simulink library "csu_ftc_final_thruster_cmd_mtv_lib"  (R2014b)
settings: Solver=ode45  StartTime=0.0  StopTime=10.0  RelTol=1e-3
undefined symbols (not defined in the file or in its folder): act_acs_cmd_duration_bias, coarse10_time, coarse11_time, coarse12_time, coarse1_time, coarse2_time, coarse3_time, coarse4_time, coarse5_time, coarse6_time, coarse7_time, coarse8_time, coarse9_time, fsw_dt
libraries: simulink x4, util_event_lib x3, util_info_lib x1
settings Model: Creator=escrane  LastModifiedBy=tgorton

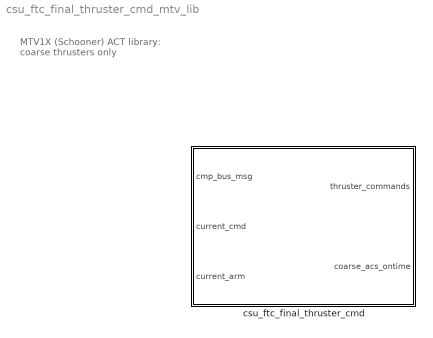
== system csu_ftc_final_thruster_cmd_mtv_lib ==
  note: MTV1X (Schooner) ACT library:
      | coarse thrusters only
  " csu_ftc_final_thruster_cmd" : Subsystem

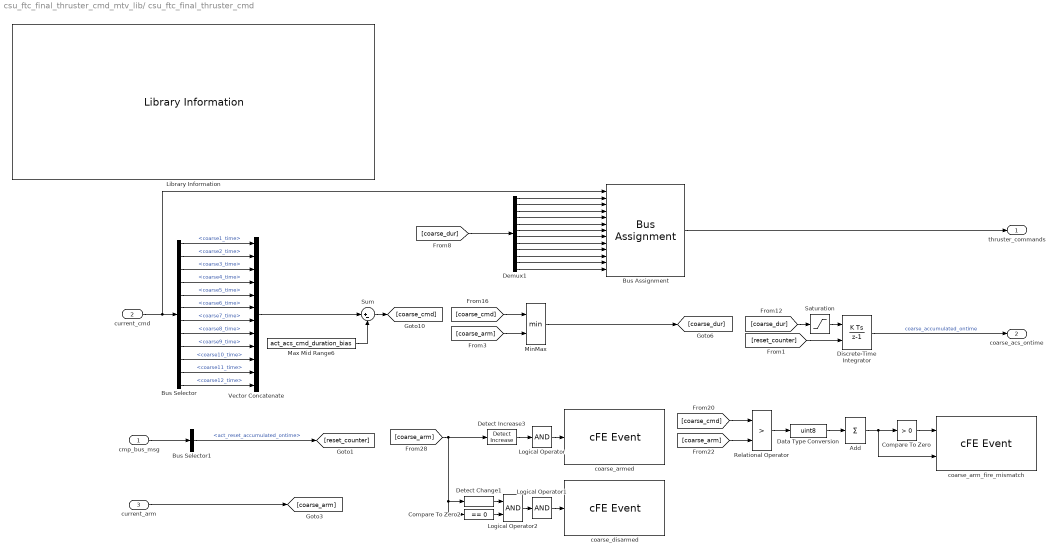
== system csu_ftc_final_thruster_cmd_mtv_lib/ csu_ftc_final_thruster_cmd ==
  cmp_bus_msg : Inport
  current_cmd : Inport  Port=2
  current_arm : Inport  Port=3
  Add : Sum  Inputs=+
  Bus Assignment : BusAssignment  AssignedSignals=coarse1_time,coarse2_time,coarse3_time,coarse4_time,coarse5_time,coarse6_time,coarse7_time,coarse8_time,coarse9_time,coarse10_time,coarse11_time,coarse12_time
  Bus Selector : BusSelector  OutputSignals=coarse1_time,coarse2_time,coarse3_time,coarse4_time,coarse5_time,coarse6_time,coarse7_time,coarse8_time,coarse9_time,coarse10_time,coarse11_time,coarse12_time
  Bus Selector1 : BusSelector  OutputSignals=act_reset_accumulated_ontime
  Compare To Zero : simulink/Logic and Bit Operations/Compare To Zero  relop=>  OutDataTypeStr=boolean
  Compare To Zero2 : simulink/Logic and Bit Operations/Compare To Zero  relop===  OutDataTypeStr=boolean
  Data Type Conversion : DataTypeConversion  OutDataTypeStr=uint8
  Demux1 : Demux  Outputs=12
  Detect Change1 : simulink/Logic and Bit Operations/Detect Change  vinit=0  InputProcessing=Inherited  OutDataTypeStr=boolean
  Detect Increase3 : simulink/Logic and Bit Operations/Detect Increase  vinit=0.0  InputProcessing=Inherited  OutDataTypeStr=boolean
  Discrete-Time Integrator : DiscreteIntegrator  gainval=1/fsw_dt  ExternalReset=rising  InitialConditionSetting=State (most efficient)  SampleTime=-1  OutDataTypeStr=uint32
  Library Information : util_info_lib/Library Information  owner='escrane'
  Logical Operator : Logic  Inputs=1  AllPortsSameDT=off  OutDataTypeStr=boolean
  Logical Operator1 : Logic  Inputs=1  AllPortsSameDT=off  OutDataTypeStr=boolean
  Logical Operator2 : Logic  AllPortsSameDT=off  OutDataTypeStr=boolean
  Max Mid Range6 : Constant  Value=act_acs_cmd_duration_bias  OutDataTypeStr=uint8
  MinMax : MinMax  Inputs=2  OutDataTypeStr=uint8
  Relational Operator : RelationalOperator  Operator=>
  Saturation : Saturate  UpperLimit=100  LowerLimit=0
  Sum : Sum  Inputs=|+-
  Vector Concatenate : Concatenate  NumInputs=12
  coarse_arm_fire_mismatch : util_event_lib/cFE Event  event_message='Coarse ACS commanded longer than enabled: %u thrusters'  event_id=19  event_severity=ERROR  event_filtered=off  event_mask=1  event_use_enums=off  event_enum_types={}
  coarse_armed : util_event_lib/cFE Event  event_message='Coarse thrusters enabled'  event_id=26  event_severity=INFORMATION  event_filtered=off  event_mask=1  event_use_enums=off  event_enum_types={}
  coarse_disarmed : util_event_lib/cFE Event  event_message='Coarse thrusters disabled'  event_id=26  event_severity=INFORMATION  event_filtered=off  event_mask=1  event_use_enums=off  event_enum_types={}
  thruster_commands : Outport
  coarse_acs_ontime : Outport  Port=2
  wires:
  Saturation/1 -> Discrete-Time Integrator/1
  Max Mid Range6/1 -> Sum/2
  Sum/1 -> [coarse_cmd]
  Logical Operator2/1 -> Logical Operator1/1
  Compare To Zero2/1 -> Logical Operator2/2
  Detect Change1/1 -> Logical Operator2/1
  Logical Operator1/1 -> coarse_disarmed/1
  Logical Operator/1 -> coarse_armed/1
  Detect Increase3/1 -> Logical Operator/1
  [coarse_arm] -> Detect Increase3/1, Detect Change1/1, Compare To Zero2/1
  Compare To Zero/1 -> coarse_arm_fire_mismatch/1
  Add/1 -> Compare To Zero/1, coarse_arm_fire_mismatch/2
  Data Type Conversion/1 -> Add/1
  Relational Operator/1 -> Data Type Conversion/1
  [coarse_arm] -> Relational Operator/2
  [coarse_cmd] -> Relational Operator/1
  [coarse_cmd] -> MinMax/1
  Vector Concatenate/1 -> Sum/1
  [coarse_dur] -> Saturation/1
  MinMax/1 -> [coarse_dur]
  current_cmd/1 -> Bus Assignment/1, Bus Selector/1
  current_arm/1 -> [coarse_arm]
  [coarse_arm] -> MinMax/2
  Bus Selector1/1 -> [reset_counter]  "<act_reset_accumulated_ontime>"
  cmp_bus_msg/1 -> Bus Selector1/1
  Discrete-Time Integrator/1 -> coarse_acs_ontime/1  "coarse_accumulated_ontime"
  [reset_counter] -> Discrete-Time Integrator/2
  Bus Selector/2 -> Vector Concatenate/2  "<coarse2_time>"
  Bus Selector/5 -> Vector Concatenate/5  "<coarse5_time>"
  Bus Selector/9 -> Vector Concatenate/9  "<coarse9_time>"
  Bus Selector/4 -> Vector Concatenate/4  "<coarse4_time>"
  Bus Selector/7 -> Vector Concatenate/7  "<coarse7_time>"
  Bus Selector/8 -> Vector Concatenate/8  "<coarse8_time>"
  Bus Selector/3 -> Vector Concatenate/3  "<coarse3_time>"
  Bus Selector/12 -> Vector Concatenate/12  "<coarse12_time>"
  Bus Selector/11 -> Vector Concatenate/11  "<coarse11_time>"
  Bus Selector/6 -> Vector Concatenate/6  "<coarse6_time>"
  Bus Selector/10 -> Vector Concatenate/10  "<coarse10_time>"
  Bus Selector/1 -> Vector Concatenate/1  "<coarse1_time>"
  [coarse_dur] -> Demux1/1
  Demux1/1 -> Bus Assignment/2
  Demux1/12 -> Bus Assignment/13
  Demux1/2 -> Bus Assignment/3
  Demux1/6 -> Bus Assignment/7
  Demux1/8 -> Bus Assignment/9
  Demux1/3 -> Bus Assignment/4
  Demux1/7 -> Bus Assignment/8
  Demux1/5 -> Bus Assignment/6
  Demux1/9 -> Bus Assignment/10
  Demux1/10 -> Bus Assignment/11
  Demux1/11 -> Bus Assignment/12
  Demux1/4 -> Bus Assignment/5
  Bus Assignment/1 -> thruster_commands/1
